simulink model "SynchGenerator_DQ_PhaseFaultAB"  (R2018a)
settings: Solver=ode23tb  StartTime=0.0  StopTime=0.3  MaxStep=200e-6  RelTol=1e-4  EnableMultiTasking=on
PreLoadFcn:
  | % Machine parameters from Kundur Examples 3.1, 3.2,  8.1 (pages 91,102, 345)
  | % "Power System Stability and Control"  McGraw-Hill  book, 1994
  | % --------------------------------------------------------------------
  | % Nominal parameters
  | Pn=  555e6;   % three-pahse nominal power (VA)
  | Vn=  24e3;    % nominal LL volatge (Vrms)
  | fn=  60;      % nominal frequency (Hz)
  | ifn= 1300;    % nominal field current (A)
  | % Note: ifn is deduced from stator-field mutual inductance Lsfd
  | %       Lsfd = Vn/sqrt(3)*sqrt(2)/ifn/wn
  | % ->     ifn = sqrt(2/3)*Vn/Lsfd/(2*pi*60)  = 1300 A
  | 
  | 
  | % Stator RL parameters (SI)
  | Rs= 0.0031;     % resistance (ohms)
  | Ll= 0.4129e-3;  % leakage inductance (H)
  | Lmd=4.5696e-3;  % d-axis magnetizing inductance (H)
  | Lmq=4.432e-3;   % q-axis magnetizing inductance (H)
  | 
  | % Field RL parameters (SI)
  | Rf= 0.0715;    %  resistance (ohms)
  | Lffd= 0.57692; %  self inductance (H)
  | % Note: Field leakage inductance Llfd wiil be later deduced from:
  | % Llfd_pu= Lffd_pu-Lmd_pu
  | 
  | % Damper RL parameters from Kundur Example 3.2
  | Rkd_pu   = 0.0284;
  | Llkd_pu  = 0.1713;
  | Rkq1_pu  = 0.00619;
  | Llkq1_pu = 0.7252;
  | Rkq2_pu  = 0.02368;
  | Llkq2_pu = 0.125;
  | 
  | % Stator base values
  | wbase=2*pi*fn;
  | Vsbase=Vn/sqrt(3)*sqrt(2);
  | Isbase=Pn/Vn/sqrt(3)*sqrt(2);
  | Zsbase=Vn^2/Pn;
  | Lsbase=Zsbase/wbase;
  | 
  | %Stator parameters in PU
  | Rs_pu=Rs/Zsbase;
  | Ll_pu=Ll/Lsbase;
  | Lmd_pu=Lmd/Lsbase;
  | Lmq_pu=Lmq/Lsbase;
  | 
  | % Field base values
  | Ifbase=ifn*Lmd_pu;
  | Vfbase=Pn/Ifbase;
  | Zfbase=Vfbase/Ifbase;
  | Lfbase=Zfbase/wbase;
  | 
  | % Transformation ratio Ns/Nf
  | Ns_Nf=2/3*Ifbase/Isbase;
  | 
  | % Field parameters in PU
  | Rf_pu=Rf/Zfbase;
  | Lffd_pu=Lffd/Lfbase;      % self inductance (pu)
  | Llfd_pu=Lffd_pu - Lmd_pu; % leakage inductance (pu)
  | Llfd= Llfd_pu*Lfbase;     % leakage inductance (H)
  | 
  | % Field parameters referred to the stator
  | Rf_prime=Rf*3/2*Ns_Nf^2;
  | Llfd_prime=Llfd*3/2*Ns_Nf^2;
  | 
  | % Nominal field voltage
  | Vfn=Rf*ifn;
  | % Nominal field voltage and current referred to stator
  | Vfn_prime=Rf_pu/Lmd_pu*Vsbase;
  | Ifn_prime=Isbase/Lmd_pu;
  | 
  | % Inertia
  | H= 3.7; % sec
  | wm= 2*pi*60; %rad/s
  | J= 2*H*Pn/wm^2; % kg.m^2
libraries: powerlib x14
Description:
  | Copyright 2008-2016 The MathWorks, Inc.
settings Model: Creator=MathWorks  LastModifiedBy=acs-mmi
settings DataIOCC: LimitDataPoints=on  SaveFormat=Array
settings OptimizationCC: ExpressionDepthLimit=2147483647  LifeSpan=inf
settings DebuggingCC: UnderspecifiedInitializationDetection=Classic  MergeDetectMultiDrivingBlocksExec=none  SolverPrmCheckMsg=warning  UnconnectedInputMsg=none  UnconnectedOutputMsg=none  UnconnectedLineMsg=none  StateNameClashWarn=warning  SFUnexpectedBacktrackingDiag=warning  SFNoUnconditionalDefaultTransitionDiag=warning  SFExecutionAtInitializationDiag=none
settings HardwareCC: ProdBitPerPointer=32  ProdBitPerSizeT=32  ProdBitPerPtrDiffT=32  ProdLargestAtomicFloat=None  ProdIntDivRoundTo=Undefined  ProdEndianess=Unspecified  ProdWordSize=32  ProdHWDeviceType=32-bit Generic
settings ModelReferenceCC: PropagateSignalLabelsOutOfModel=off
settings CodeAppCC: StateflowObjectComments=on
settings GRTTargetCC: TargetLangStandard=C89/C90 (ANSI)  GeneratePreprocessorConditionals=Disable all
settings ConfigComp: CovMetricSettings=dw  CovHtmlReporting=on  CovSaveCumulativeToWorkspaceVar=on  CovSaveSingleToWorkspaceVar=on  CovExternalEMLEnable=off  CovSFcnEnable=off
settings SimscapeCC: SimscapeNormalizeSystem=off

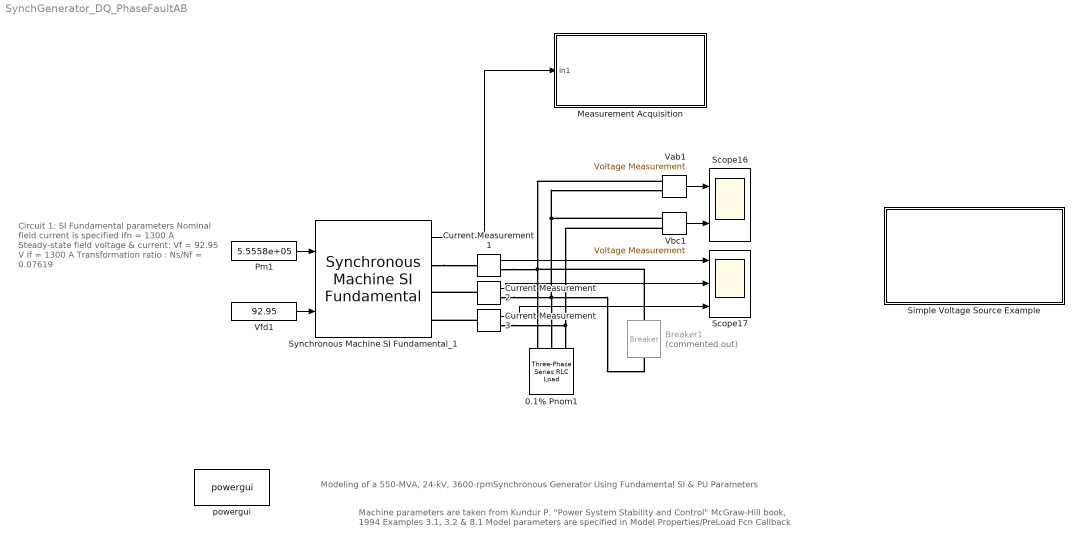
== system SynchGenerator_DQ_PhaseFaultAB ==
  note: Circuit 1: SI Fundamental parameters
      |
      | Nominal field current is specified
      |      ifn = 1300 A
      | Steady-state field voltage & current:
      |     Vf = 92.95 V
      |     If  = 1300 A
      | Transformation ratio :
      |     Ns/Nf = 0.07619
  note: Machine parameters are taken from Kundur P.  "Power System Stability and Control" McGraw-Hill  book, 1994 Examples 3.1, 3.2 &  8.1
      | Model parameters are specified  in Model Properties/PreLoad Fcn Callback
  note: Modeling of a 550-MVA, 24-kV, 3600-rpmSynchronous Generator Using Fundamental SI & PU Parameters
  0.1% Pnom1 : powerlib/Elements/Three-Phase Series RLC Load  LConnTagsString=A|B|C  Configuration=Y (grounded)  NominalVoltage=24e3  Vabc=[1e3 1e3 1e3]  Vabcp=[1e3 1e3 1e3]  NominalFrequency=60  UnbalancedPower=off  ActivePower=555e6/1e3  InductivePower=0  CapacitivePower=0  Pabc=[10e3 9e3 11e3]  QLabc=[100 90 110]  QCabc=[100 90 110]  Pabcp=[10e3 9e3 11e3]  QLabcp=[100 90 110]  QCabcp=[100 90 110]  Measurements=Branch voltages and currents  LoadType=constant Z
  Breaker1 : powerlib/Elements/Breaker  Commented=on  InitialState=0  SwitchingTimes=[ 0.1 0.2 ]  External=off  BreakerResistance=0.01  SnubberResistance=1e6  SnubberCapacitance=inf  Measurements=None  MoreParameters=off  NoBreakLoop=off
      settings: SourceProductName=Simscape Power Systems
  Current Measurement1 : powerlib/Measurements/Current Measurement  PhasorSimulation=off  OutputType=Complex  PSBequivalent=0
  Current Measurement2 : powerlib/Measurements/Current Measurement  PhasorSimulation=off  OutputType=Complex  PSBequivalent=0
  Current Measurement3 : powerlib/Measurements/Current Measurement  PhasorSimulation=off  OutputType=Complex  PSBequivalent=0
  Measurement Acquisition : Subsystem
  Pm1 : Constant  Value=5.5558e+05
  Scope16 : Scope  NumInputPorts=2
  Scope17 : Scope  NumInputPorts=3
  Simple Voltage Source Example : Subsystem
  Synchronous Machine SI Fundamental_1 : powerlib/Machines/Synchronous Machine SI Fundamental  PresetModel=No  MechanicalLoad=Mechanical power Pm  ShowDetailedParameters=on  RotorType=Round  Units=SI fundamental parameters  MeasurementBus=off  NominalParameters="[ Pn  Vn    fn  ifn ]"  Stator="[ Rs    Ll    Lmd     Lmq ]"  Field="[Rf   Llfd ]*3/2*(Ns_Nf)^2"  Dampers2="[Rkd_pu Llkd_pu  Rkq1_pu  Llkq1_pu Rkq2_pu  Llkq2_pu ] .*[Zsbase  Lsbase  Zsbase  Lsbase  Zsbase  Lsbase]"  Dampers1="[Rkd_pu  Llkd_pu  Rkq1_pu  Llkq1_pu].*[Zsbase  Lsbase  Zsbase  Lsbase]"  Mechanical="[ J  0 1 ]"  PolePairs=1  InitialConditions=[0 -89.8991 18.9011 18.9011 18.9011 4.052e-12 -120 120 92.9504]  SetSaturation=off  Saturation=[695.64,774.7,917.5,1001.6,1082.2,1175.9,1293.6,1430.2,1583.7;9660,10623,12243,13063,13757,14437,15180,15890,16567]  DisplayVfd=off  LoadFlowParameters=[1,0,0,0,0]  TsPowergui=0  TsBlock=-1  IterativeModel=Trapezoidal iterative (alg. loop)  IterativeDiscreteModel=Trapezoidal non iterative  BusType=swing  Pref=0  Qref=0  Qmin=-inf  Qmax=inf  PLF=0  QLF=0
      settings: SourceProductName=Simscape Power Systems  SourceProductBaseCode=PS
  Vab1 : powerlib/Measurements/Voltage Measurement  PhasorSimulation=off  OutputType=Complex  PSBequivalent=0
  Vbc1 : powerlib/Measurements/Voltage Measurement  PhasorSimulation=off  OutputType=Complex  PSBequivalent=0
  Vfd1 : Constant  Value=92.95
  powergui : powerlib/powergui  Priority=1  SimulationMode=Continuous  SampleTime=50e-6  frequency=60  Iterations=50  frequencyindice=60  Pbase=100e6  ErrMax=0.0001  UnitsV=kV  UnitsW=MW  buscounter=0  FunctionMessages=off  echomessages=off  EnableUseOfTLC=off  CurrentSourceSwitches=off  DisableSnubberDevices=on  DisableRonSwitches=off  DisableVfSwitches=off  DisplayEquations=off  SolverType=Tustin  Interpol=off  ExternalGateDelay=off  methode=off  Ts=0  x0status=blocks  SPID=on  SwTol=0  HookPort=off  RestoreLinks=warning  ResistiveCurrentMeasurement=off  Frange=[0:2:500]  Ylog=off  Xlog=on  ShowGrid=off  save=off  variable=ZData  structure=0  ZoomFFT=off  StartTime=0.0  cycles=1  DisplayStyle=1  fundamental=60  FreqAxis=off  MaxFrequency=1000  frequencyindicesteady=1  RmsSteady=1  display=off
  wires:
  Pm1/1 -> Synchronous Machine SI Fundamental_1/1
  Vfd1/1 -> Synchronous Machine SI Fundamental_1/2
  Vab1/1 -> Scope16/1
  Current Measurement1/1 -> Scope17/1
  Vbc1/1 -> Scope16/2
  Current Measurement2/1 -> Scope17/2
  Current Measurement3/1 -> Scope17/3
  Synchronous Machine SI Fundamental_1/1 -> Measurement Acquisition/1(In1)
  connections:
  Vbc1/LConn2 -- Current Measurement3/RConn1 -- 0.1% Pnom1/LConn3
  Current Measurement2/RConn1 -- Breaker1/RConn1 -- 0.1% Pnom1/LConn2 -- Vbc1/LConn1 -- Vab1/LConn2
  Synchronous Machine SI Fundamental_1/RConn1 -- Current Measurement1/LConn1
  Current Measurement1/RConn1 -- Breaker1/LConn1 -- Vab1/LConn1 -- 0.1% Pnom1/LConn1
  Current Measurement2/LConn1 -- Synchronous Machine SI Fundamental_1/RConn2
  Current Measurement3/LConn1 -- Synchronous Machine SI Fundamental_1/RConn3

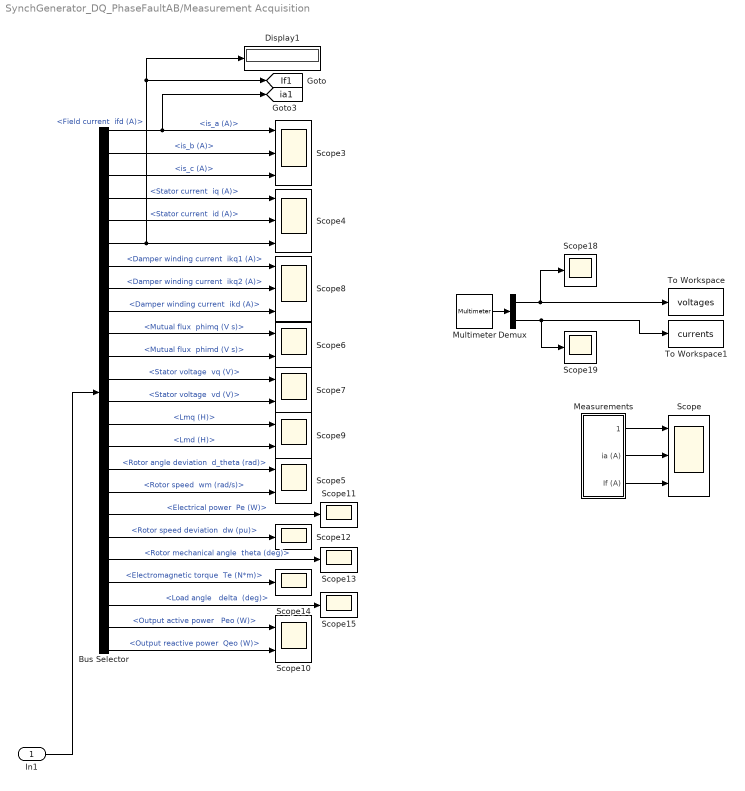
== system SynchGenerator_DQ_PhaseFaultAB/Measurement Acquisition ==
  In1 : Inport
  Bus Selector : BusSelector  OutputSignals="Stator current.is_a (A),Stator current.is_b (A),Stator current.is_c (A),dq0 components.Stator current  iq (A),dq0 components.Stator current  id (A),dq0 components.Field current  ifd (A),dq0 components.Damper winding current  ikq1 (A),dq0 components.Damper winding current  ikq2 (A),dq0 components.Damper winding current  ikd (A),dq0 components.Mutual flux  phimq (V s),dq0 components.Mutual flux  phimd (V s),dq0 components.Stator voltage  vq (V),dq0 components.Stator voltage  vd (V),dq0 components.Lmq (H),dq0 components.Lmd (H),Mechanical.Rotor angle deviation  d_theta (rad),Mechanical.Rotor speed  wm (rad/s),Mechanical.Electrical power  Pe (W),Mechanical.Rotor speed deviation  dw (pu),Mechanical.Rotor mechanical angle  theta (deg),Mechanical.Electromagnetic torque  Te (N*m),Load angle   delta  (deg),Output active power   Peo (W),Output reactive power  Qeo (W)"
  Demux : Demux  Outputs=2
  Display1 : Display
  Measurements : Subsystem
  Multimeter : powerlib/Measurements/Multimeter  PhasorSimulation=off  OutputType=Complex  sel=[1 2 3 4 5 6]  L=6  Gain=[1 1 1 1 1 1]  yselected={'Uag: 0.1% Pnom1','Ubg: 0.1% Pnom1','Ucg: 0.1% Pnom1','Iag: 0.1% Pnom1','Ibg: 0.1% Pnom1','Icg: 0.1% Pnom1'};  PSBOutputType=1  PSBequivalent=0  AxesSetting=[0,0.1,-100,100]  Display=0  SavedBlockNames=-11
  Scope{,3..4,8} (4 alike) : Scope  NumInputPorts=3
  Scope{5..7,9..10} (5 alike) : Scope  NumInputPorts=2
  Scope{11..15,18..19} (7 alike) : Scope
  To Workspace : ToWorkspace  VariableName=voltages  SaveFormat=Timeseries  SampleTime=-1
  To Workspace1 : ToWorkspace  VariableName=currents  SaveFormat=Timeseries  SampleTime=-1
  tag scope: If1=global, ia1=global
  wires:
  Bus Selector/20 -> Scope13/1  "<Rotor mechanical angle  theta (deg)>"
  Bus Selector/18 -> Scope11/1  "<Electrical power  Pe (W)>"
  Measurements/2(ia (A)) -> Scope/2
  Bus Selector/3 -> Scope3/3  "<is_c (A)>"
  Bus Selector/14 -> Scope9/1  "<Lmq (H)>"
  Demux/2 -> To Workspace1/1, Scope19/1
  Bus Selector/6 -> Scope4/3, Display1/1, [If1]  "<Field current  ifd (A)>"
  Bus Selector/16 -> Scope5/1  "<Rotor angle deviation  d_theta (rad)>"
  Bus Selector/21 -> Scope14/1  "<Electromagnetic torque  Te (N*m)>"
  Bus Selector/1 -> [ia1], Scope3/1  "<is_a (A)>"
  Bus Selector/19 -> Scope12/1  "<Rotor speed deviation  dw (pu)>"
  Bus Selector/2 -> Scope3/2  "<is_b (A)>"
  Bus Selector/12 -> Scope7/1  "<Stator voltage  vq (V)>"
  Bus Selector/4 -> Scope4/1  "<Stator current  iq (A)>"
  Bus Selector/8 -> Scope8/2  "<Damper winding current  ikq2 (A)>"
  Bus Selector/10 -> Scope6/1  "<Mutual flux  phimq (V s)>"
  In1/1 -> Bus Selector/1
  Bus Selector/17 -> Scope5/2  "<Rotor speed  wm (rad/s)>"
  Bus Selector/5 -> Scope4/2  "<Stator current  id (A)>"
  Measurements/1(Vab (pu)) -> Scope/1
  Bus Selector/15 -> Scope9/2  "<Lmd (H)>"
  Bus Selector/22 -> Scope15/1  "<Load angle   delta  (deg)>"
  Bus Selector/23 -> Scope10/1  "<Output active power   Peo (W)>"
  Bus Selector/7 -> Scope8/1  "<Damper winding current  ikq1 (A)>"
  Bus Selector/9 -> Scope8/3  "<Damper winding current  ikd (A)>"
  Bus Selector/11 -> Scope6/2  "<Mutual flux  phimd (V s)>"
  Demux/1 -> To Workspace/1, Scope18/1
  Multimeter/1 -> Demux/1
  Bus Selector/24 -> Scope10/2  "<Output reactive power  Qeo (W)>"
  Measurements/3(If (A)) -> Scope/3
  Bus Selector/13 -> Scope7/2  "<Stator voltage  vd (V)>"

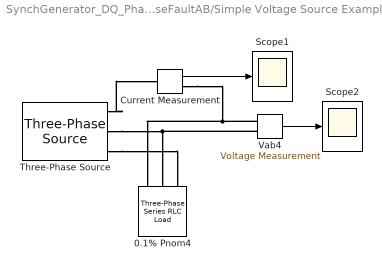
== system SynchGenerator_DQ_PhaseFaultAB/Simple Voltage Source Example ==
  0.1% Pnom4 : powerlib/Elements/Three-Phase Series RLC Load  LConnTagsString=A|B|C  Configuration=Y (grounded)  NominalVoltage=24e3  Vabc=[1e3 1e3 1e3]  Vabcp=[1e3 1e3 1e3]  NominalFrequency=60  UnbalancedPower=off  ActivePower=555e6/1e3  InductivePower=0  CapacitivePower=0  Pabc=[10e3 9e3 11e3]  QLabc=[100 90 110]  QCabc=[100 90 110]  Pabcp=[10e3 9e3 11e3]  QLabcp=[100 90 110]  QCabcp=[100 90 110]  Measurements=None  LoadType=constant Z
  Current Measurement : powerlib/Measurements/Current Measurement  PhasorSimulation=off  OutputType=Complex  PSBequivalent=0
  Scope1 : Scope
  Scope2 : Scope
  Three-Phase Source : powerlib/Electrical Sources/Three-Phase Source  InternalConnection=Yg  VoltagePhases=off  Voltage=24e3  PhaseAngle=0  Voltage_phases=[25e3 25e3 25e3]/sqrt(3)  PhaseAngles_phases=[0 -120 +120]  Frequency=60  NonIdealSource=off  SpecifyImpedance=off  Resistance=0  Inductance=0  ShortCircuitLevel=100e6  BaseVoltage=25e3  XRratio=7  BusType=swing  Pref=10e3  Qref=0  Prefabc=[10e3, 10e3, 10e3]  Qrefabc=[0, 0, 0]  Qmin=-inf  Qmax=inf
  Vab4 : powerlib/Measurements/Voltage Measurement  PhasorSimulation=off  OutputType=Complex  PSBequivalent=0
  wires:
  Vab4/1 -> Scope2/1
  Current Measurement/1 -> Scope1/1
  connections:
  Current Measurement/RConn1 -- Vab4/LConn1 -- 0.1% Pnom4/LConn1
  Three-Phase Source/RConn3 -- 0.1% Pnom4/LConn3
  Three-Phase Source/RConn2 -- Vab4/LConn2 -- 0.1% Pnom4/LConn2
  Three-Phase Source/RConn1 -- Current Measurement/LConn1

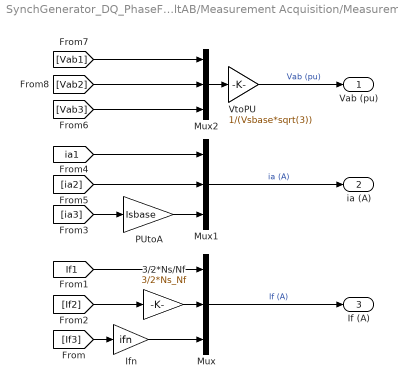
== system SynchGenerator_DQ_PhaseFaultAB/Measurement Acquisition/Measurements ==
  3/2*Ns/Nf : Gain  Gain=3/2*Ns_Nf
  Ifn : Gain  Gain=ifn
  Mux : Mux  Inputs=3
  Mux1 : Mux  Inputs=3
  Mux2 : Mux  Inputs=3
  PUtoA : Gain  Gain=Isbase
  VtoPU : Gain  Gain=1/(Vsbase*sqrt(3))
  Vab (pu) : Outport
  ia (A) : Outport  Port=2
  If (A) : Outport  Port=3
  wires:
  [Vab2] -> Mux2/2
  [Vab1] -> Mux2/1
  Mux2/1 -> VtoPU/1
  VtoPU/1 -> Vab (pu)/1  "Vab (pu)"
  [ia2] -> Mux1/2
  [Vab3] -> Mux2/3
  PUtoA/1 -> Mux1/3
  Ifn/1 -> Mux/3
  Mux/1 -> If (A)/1  "If (A)"
  [ia3] -> PUtoA/1
  [If3] -> Ifn/1
  [If2] -> 3/2*Ns/Nf/1
  Mux1/1 -> ia (A)/1  "ia (A)"
  3/2*Ns/Nf/1 -> Mux/2
  [If1] -> Mux/1
  [ia1] -> Mux1/1
